simulink model "Multiphase"  (R2018b)
settings: Solver=FixedStepDiscrete  StartTime=0.0  StopTime=10.0  FixedStep=0.05  RelTol=1e-3  EnableMultiTasking=on
undefined symbols (not defined in the file): HRTIM_ADC1R_AD1TAC2, HRTIM_ADC1R_AD1TBC2, HRTIM_ADC1R_AD1TCC2, HRTIM_ADC1R_AD1TDC3, HRTIM_ADC1R_AD1TDC4, HRTIM_TIMERINDEX_TIMER_D, sTimerxRegs
libraries: HRTIMERS_Lib x9, GPIO_Lib x9, REG_Lib x8, STM32_Config_Lib x1
settings Model: Creator=reynaudp  LastModifiedBy=bannou
settings DataIOCC: LimitDataPoints=on  SaveFormat=Array
settings OptimizationCC: DefaultParameterBehavior=Inlined  LifeSpan=1
settings DebuggingCC: SolverPrmCheckMsg=warning  MultiTaskDSMMsg=none  AllowSymbolicDim=off  SFUnexpectedBacktrackingDiag=warning  SFNoUnconditionalDefaultTransitionDiag=warning  SFExecutionAtInitializationDiag=none
settings HardwareCC: ProdBitPerPointer=32  ProdBitPerSizeT=32  ProdBitPerPtrDiffT=32  ProdLargestAtomicInteger=Integer  ProdWordSize=32  ProdHWDeviceType=STMicroelectronics->STM32 32-bit Cortex-M
settings ModelReferenceCC: PropagateSignalLabelsOutOfModel=off
settings SFSimCC: SimUseLocalCustomCode=off  MATLABDynamicMemAlloc=off
settings RTWCC: SystemTargetFile=stm32.tlc  TemplateMakefile=stm32.tmf  Description=stm32 (Embedded Target)  GenerateReport=on  RTWUseLocalCustomCode=off
settings CodeAppCC: IgnoreCustomStorageClasses=off  CustomSymbolStrType=$N$R$M  SimulinkBlockComments=off
settings STFCustomTargetCC: CodeReplacementLibrary=ARM CMSIS SIN COS  ParMdlRefBuildCompliant=on  IncludeMdlTerminateFcn=off  CombineOutputUpdateFcns=on  ERTCustomFileBanners=on  SupportNonFinite=off  SupportComplex=off  SupportContinuousTime=off  SupportNonInlinedSFcns=off  RemoveResetFunc=on  MATLABClassNameForMDSCustomization=Simulink.SoftwareTarget.ERTCustomization  SystemTargetFile=stm32.tlc
settings ERTTargetCC: CodeReplacementLibrary=ARM CMSIS SIN COS  MultiwordLength=2048  CompOptLevelCompliant=off  ConcurrentExecutionCompliant=off  IncludeMdlTerminateFcn=off  SupportNonFinite=off  SupportComplex=off  ModelStepFunctionPrototypeControlCompliant=off  CPPClassGenCompliant=off  UseToolchainInfoCompliant=off  ERTSrcFileBannerTemplate=sourceFileTemplate.cgt  ERTHdrFileBannerTemplate=sourceFileTemplate.cgt  ERTDataSrcFileTemplate=sourceFileTemplate.cgt  ERTDataHdrFileTemplate=sourceFileTemplate.cgt  ERTCustomFileTemplate=customRoutineProcess.tlc  ConvertIfToSwitch=off  SuppressUnreachableDefaultCases=off
settings ConfigComp: CovMetricSettings=dw  CovHtmlReporting=on  CovSaveCumulativeToWorkspaceVar=on  CovSaveSingleToWorkspaceVar=on  CovExternalEMLEnable=off  CovSFcnEnable=off

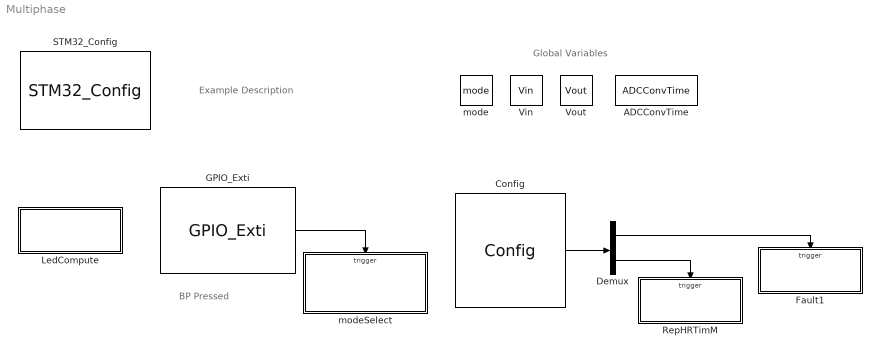
== system Multiphase ==
  note: Example Description
  note: BP Pressed
  note: Global Variables
  ADCConvTime : DataStoreMemory  DataStoreName=ADCConvTime  ReadBeforeWriteMsg=warning  WriteAfterWriteMsg=warning  WriteAfterReadMsg=warning  InitialValue=1152  ShowAdditionalParam=off  OutDataTypeStr=uint32
  Config : HRTIMERS_Lib/Config  currentHRTIM=HRTIM1  NbHRTim=1  HRTIM_Name=HRTIM1  HRTIM_Clock=144000000  TIM_IRQ_F1=on  TIM_IRQ_F2=off  TIM_IRQ_F3=off  TIM_IRQ_F4=off  TIM_IRQ_F5=off  TIM_IRQ_F6=off  TIM_IRQ_SF=off  TIM_IRQ_BMP=off  TIM_IRQ_DLLCALL=off  TIM_IRQ_SYNC=off  TIM_IRQ_BURST_DMA=off  TIM_IRQ_DMA_ERR=off  M_DMA=off  M_IT_global=on  M_Tim_div=MUL32  M_Period=40960  M_PWM_Period=112500  M_Unit1=8192  M_Unit2=16384  M_Unit3=24576  M_Unit4=32768  TIM_IRQ_UPDM=off  TIM_IRQ_REPM=on  TIM_IRQ_COMP1=off  TIM_IRQ_COMP2=off  TIM_IRQ_COMP3=off  TIM_IRQ_COMP4=off  A_Mode=Advanced  A_DMA=off  A_IT_global=off  A_Tim_div=MUL32  A_Period=39807  A_PWM_Period=115759  A_Capture1=off  A_Capture2=off  TA1_Enable=off  TA1_Polarity=HIGH  TA1_Chopper=off  TA2_Enable=on  TA2_Polarity=HIGH  TA2_Chopper=off  A_Unit1=4096  A_Unit2=2048  A_Unit3=37503  A_Unit4=38655  A_Output_Comp1=off  A_Comp_Polarity1=HIGH  A_CompVal1=0  A_Output_Comp2=off  A_Comp_Polarity2=HIGH  A_CompVal2=0  A_Output_PWM1=off  A_Output_Polarity1=HIGH  A_DutyVal1=0  A_DutyIn1=off  A_Output_PWM2=off  A_Output_Polarity2=HIGH  A_DutyVal2=0  A_DutyIn2=off  A_OnePulse1=off  A_OnePulse_Polarity1=HIGH  A_OnePulse_CompVal1=0  A_OnePulse2=off  A_OnePulse_Polarity2=HIGH  A_OnePulse_CompVal2=0  TIM_IRQ_UPDA=off  TIM_IRQ_REPA=off  TIM_IRQ_COMP1A=off  TIM_IRQ_COMP2A=off  TIM_IRQ_COMP3A=off  TIM_IRQ_COMP4A=off  TIM_IRQ_CAPT1A=off  TIM_IRQ_CAPT2A=off  TIM_IRQ_DELA=off  TIM_IRQ_RESET_CPTA=off  TIM_IRQ_OUT1SA=off  TIM_IRQ_OUT1RA=off  TIM_IRQ_OUT2SA=off  TIM_IRQ_OUT2RA=off  B_Mode=Advanced  B_DMA=off  B_IT_global=off  B_Tim_div=MUL32  B_Period=39807  B_PWM_Period=115759  B_Capture1=off  B_Capture2=off  TB1_Enable=on  TB1_Polarity=HIGH  TB1_Chopper=off  TB2_Enable=off  TB2_Polarity=HIGH  TB2_Chopper=off  B_Unit1=4096  B_Unit2=2048  B_Unit3=19327  B_Unit4=18175  B_Output_Comp1=off  B_Comp_Polarity1=HIGH  B_CompVal1=0  B_Output_Comp2=off  B_Comp_Polarity2=HIGH  B_CompVal2=0  B_Output_PWM1=off  B_Output_Polarity1=HIGH  B_DutyVal1=0  B_DutyIn1=off  B_Output_PWM2=off  B_Output_Polarity2=HIGH  B_DutyVal2=0  B_DutyIn2=off  B_OnePulse1=off  B_OnePulse_Polarity1=HIGH  B_OnePulse_CompVal1=0  B_OnePulse2=off  B_OnePulse_Polarity2=HIGH  B_OnePulse_CompVal2=0  TIM_IRQ_UPDB=off  TIM_IRQ_REPB=off  TIM_IRQ_COMP1B=off  TIM_IRQ_COMP2B=off  TIM_IRQ_COMP3B=off  TIM_IRQ_COMP4B=off  TIM_IRQ_CAPT1B=off  TIM_IRQ_CAPT2B=off  TIM_IRQ_DELB=off  TIM_IRQ_RESET_CPTB=off  TIM_IRQ_OUT1SB=off  TIM_IRQ_OUT1RB=off  TIM_IRQ_OUT2SB=off  TIM_IRQ_OUT2RB=off  C_Mode=Advanced  C_DMA=off  C_IT_global=off  C_Tim_div=MUL32  C_Period=39807  C_PWM_Period=115759  C_Capture1=off  C_Capture2=off  TC1_Enable=off  TC1_Polarity=HIGH  TC1_Chopper=off  TC2_Enable=on  TC2_Polarity=HIGH  TC2_Chopper=off  C_Unit1=4096  C_Unit2=2048  C_Unit3=12500  C_Unit4=11348  C_Output_Comp1=off  C_Comp_Polarity1=HIGH  C_CompVal1=0  C_Output_Comp2=off  C_Comp_Polarity2=HIGH  C_CompVal2=0  C_Output_PWM1=off  C_Output_Polarity1=HIGH  C_DutyVal1=0  C_DutyIn1=off  C_Output_PWM2=off  C_Output_Polarity2=HIGH  C_DutyVal2=0  C_DutyIn2=off  C_OnePulse1=off  C_OnePulse_Polarity1=HIGH  C_OnePulse_CompVal1=0  C_OnePulse2=off  C_OnePulse_Polarity2=HIGH  C_OnePulse_CompVal2=0  TIM_IRQ_UPDC=off  TIM_IRQ_REPC=off  TIM_IRQ_COMP1C=off  TIM_IRQ_COMP2C=off  TIM_IRQ_COMP3C=off  TIM_IRQ_COMP4C=off  TIM_IRQ_CAPT1C=off  TIM_IRQ_CAPT2C=off  TIM_IRQ_DELC=off  TIM_IRQ_RESET_CPTC=off  TIM_IRQ_OUT1SC=off  TIM_IRQ_OUT1RC=off  TIM_IRQ_OUT2SC=off  TIM_IRQ_OUT2RC=off  D_Mode=Advanced  D_DMA=off  D_IT_global=off  D_Tim_div=MUL32  D_Period=39807  D_PWM_Period=115759  D_Capture1=off  D_Capture2=off  TD1_Enable=on  TD1_Polarity=HIGH  TD1_Chopper=off  TD2_Enable=on  TD2_Polarity=HIGH  TD2_Chopper=off  D_Unit1=4096  D_Unit2=12288  D_Unit3=2048  D_Unit4=10240  D_Output_Comp1=off  D_Comp_Polarity1=HIGH  D_CompVal1=0  D_Output_Comp2=off  D_Comp_Polarity2=HIGH  D_CompVal2=0  D_Output_PWM1=off  D_Output_Polarity1=HIGH  D_DutyVal1=0  D_DutyIn1=off  D_Output_PWM2=off  D_Output_Polarity2=HIGH  D_DutyVal2=0  D_DutyIn2=off  D_OnePulse1=off  D_OnePulse_Polarity1=HIGH  D_OnePulse_CompVal1=0  D_OnePulse2=off  D_OnePulse_Polarity2=HIGH  D_OnePulse_CompVal2=0  TIM_IRQ_UPDD=off  TIM_IRQ_REPD=off  TIM_IRQ_COMP1D=off  TIM_IRQ_COMP2D=off  TIM_IRQ_COMP3D=off  TIM_IRQ_COMP4D=off  TIM_IRQ_CAPT1D=off  TIM_IRQ_CAPT2D=off  TIM_IRQ_DELD=off  TIM_IRQ_RESET_CPTD=off  TIM_IRQ_OUT1SD=off  TIM_IRQ_OUT1RD=off  TIM_IRQ_OUT2SD=off  TIM_IRQ_OUT2RD=off  E_Mode=Advanced  E_DMA=off  E_IT_global=off  E_Tim_div=MUL32  E_Period=0  E_PWM_Period=Inf  E_Capture1=off  E_Capture2=off  TE1_Enable=off  TE1_Polarity=HIGH  TE1_Chopper=off  TE2_Enable=off  TE2_Polarity=HIGH  TE2_Chopper=off  E_Unit1=0  E_Unit2=0  E_Unit3=0  E_Unit4=0  E_Output_Comp1=off  E_Comp_Polarity1=HIGH  E_CompVal1=0  E_Output_Comp2=off  E_Comp_Polarity2=HIGH  E_CompVal2=0  E_Output_PWM1=off  E_Output_Polarity1=HIGH  E_DutyVal1=0  E_DutyIn1=off  E_Output_PWM2=off  E_Output_Polarity2=HIGH  E_DutyVal2=0  E_DutyIn2=off  E_OnePulse1=off  E_OnePulse_Polarity1=HIGH  E_OnePulse_CompVal1=0  E_OnePulse2=off  E_OnePulse_Polarity2=HIGH  E_OnePulse_CompVal2=0  TIM_IRQ_UPDE=off  TIM_IRQ_REPE=off  TIM_IRQ_COMP1E=off  TIM_IRQ_COMP2E=off  TIM_IRQ_COMP3E=off  TIM_IRQ_COMP4E=off  TIM_IRQ_CAPT1E=off  TIM_IRQ_CAPT2E=off  TIM_IRQ_DELE=off  TIM_IRQ_RESET_CPTE=off  TIM_IRQ_OUT1SE=off  TIM_IRQ_OUT1RE=off  TIM_IRQ_OUT2SE=off  TIM_IRQ_OUT2RE=off  F_Mode=Advanced  F_DMA=off  F_IT_global=off  F_Tim_div=MUL32  F_Period=0  F_PWM_Period=Inf  F_Capture1=off  F_Capture2=off  TF1_Enable=off  TF1_Polarity=HIGH  TF1_Chopper=off  TF2_Enable=off  TF2_Polarity=HIGH  TF2_Chopper=off  F_Unit1=0  F_Unit2=0  F_Unit3=0  F_Unit4=0  F_Output_Comp1=off  F_Comp_Polarity1=HIGH  F_CompVal1=0  F_Output_Comp2=off  F_Comp_Polarity2=HIGH  F_CompVal2=0  F_Output_PWM1=off  F_Output_Polarity1=HIGH  F_DutyVal1=0  F_DutyIn1=off  F_Output_PWM2=off  F_Output_Polarity2=HIGH  F_DutyVal2=0  F_DutyIn2=off  F_OnePulse1=off  F_OnePulse_Polarity1=HIGH  F_OnePulse_CompVal1=0  F_OnePulse2=off  F_OnePulse_Polarity2=HIGH  F_OnePulse_CompVal2=0  TIM_IRQ_UPDF=off  TIM_IRQ_REPF=off  TIM_IRQ_COMP1F=off  TIM_IRQ_COMP2F=off  TIM_IRQ_COMP3F=off  TIM_IRQ_COMP4F=off  TIM_IRQ_CAPT1F=off  TIM_IRQ_CAPT2F=off  TIM_IRQ_DELF=off  TIM_IRQ_RESET_CPTF=off  TIM_IRQ_OUT1SF=off  TIM_IRQ_OUT1RF=off  TIM_IRQ_OUT2SF=off  TIM_IRQ_OUT2RF=off  M_Used=on  A_Used=on  B_Used=on  C_Used=on  D_Used=on  E_Used=off  F_Used=off
      settings: SourceProductName=Target Support Package - STM32 Adapter
  Demux : Demux  Outputs=2
  Fault1 : Subsystem  TreatAsAtomicUnit=on
  GPIO_Exti : GPIO_Lib/GPIO_Exti  Priority=0  Port_name=GPIOA  Pin_0=on  Pin_1=off  Pin_2=off  Pin_3=off  Pin_4=off  Pin_5=off  Pin_6=off  Pin_7=off  Pin_8=off  Pin_9=off  Pin_10=off  Pin_11=off  Pin_12=off  Pin_13=off  Pin_14=off  Pin_15=off  PinList=GPIOA0
      settings: SourceProductName=Target Support Package - STM32 Adapter
  LedCompute : Subsystem
  RepHRTimM : Subsystem  TreatAsAtomicUnit=on
  STM32_Config : STM32_Config_Lib/STM32_Config  Priority=0  Project_Path=.\  Config_File=Multiphase.ioc  MCU_Name=STM32F334C8Tx
      settings: SourceProductName=Target Support Package - STM32 Adapter
  Vin : DataStoreMemory  DataStoreName=Vin  ReadBeforeWriteMsg=warning  WriteAfterWriteMsg=warning  WriteAfterReadMsg=warning  ShowAdditionalParam=off  OutMin=0  OutMax=5000  OutDataTypeStr=uint32
  Vout : DataStoreMemory  DataStoreName=Vout  ReadBeforeWriteMsg=warning  WriteAfterWriteMsg=warning  WriteAfterReadMsg=warning  ShowAdditionalParam=off  OutMin=0  OutDataTypeStr=uint32
  mode : DataStoreMemory  DataStoreName=mode  ReadBeforeWriteMsg=warning  WriteAfterWriteMsg=warning  WriteAfterReadMsg=warning  InitialValue=6  ShowAdditionalParam=off  OutMin=0  OutMax=12  OutDataTypeStr=uint8
  modeSelect : Subsystem  TreatAsAtomicUnit=on
  wires:
  GPIO_Exti/1 -> modeSelect/Trigger
  Config/1 -> Demux/1
  Demux/1 -> Fault1/Trigger
  Demux/2 -> RepHRTimM/Trigger

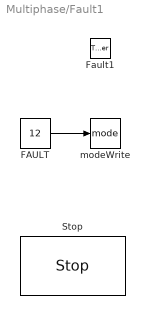
== system Multiphase/Fault1 ==
  Fault1 : TriggerPort  TriggerType=function-call  VariantControl=Variant
  FAULT : Constant  Value=12  OutDataTypeStr=uint8
  Stop : HRTIMERS_Lib/Stop  currentHRTIM=HRTIM1  NbHRTim=1  HRTIM_Name=HRTIM1  TA1_Stop=off  TA2_Stop=on  TB1_Stop=on  TB2_Stop=off  TC1_Stop=off  TC2_Stop=on  TD1_Stop=on  TD2_Stop=on  TE1_Stop=off  TE2_Stop=off  TF1_Stop=off  TF2_Stop=off
      settings: SourceProductName=Target Support Package - STM32 Adapter
  modeWrite : DataStoreWrite  DataStoreName=mode
  wires:
  FAULT/1 -> modeWrite/1

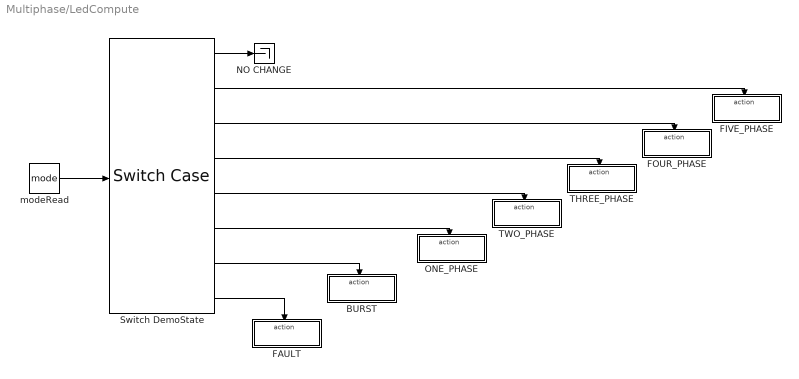
== system Multiphase/LedCompute ==
  BURST : Subsystem  TreatAsAtomicUnit=on
  FAULT : Subsystem  TreatAsAtomicUnit=on
  FIVE_PHASE : Subsystem  TreatAsAtomicUnit=on
  FOUR_PHASE : Subsystem  TreatAsAtomicUnit=on
  NO CHANGE : Terminator
  ONE_PHASE : Subsystem  TreatAsAtomicUnit=on
  Switch DemoState : SwitchCase  CaseConditions={[0,5],6,7,8,9,10,11,12}  ShowDefaultCase=off
  THREE_PHASE : Subsystem  TreatAsAtomicUnit=on
  TWO_PHASE : Subsystem  TreatAsAtomicUnit=on
  modeRead : DataStoreRead  DialogController=Simulink.DDGSource  DataStoreName=mode
  wires:
  modeRead/1 -> Switch DemoState/1
  Switch DemoState/2 -> FIVE_PHASE/Action
  Switch DemoState/3 -> FOUR_PHASE/Action
  Switch DemoState/4 -> THREE_PHASE/Action
  Switch DemoState/5 -> TWO_PHASE/Action
  Switch DemoState/6 -> ONE_PHASE/Action
  Switch DemoState/7 -> BURST/Action
  Switch DemoState/8 -> FAULT/Action
  Switch DemoState/1 -> NO CHANGE/1

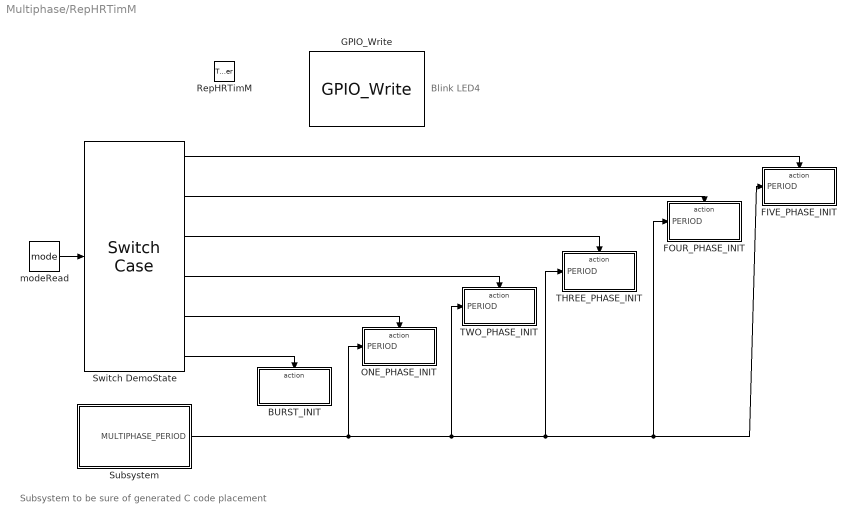
== system Multiphase/RepHRTimM ==
  note: Blink LED4
  note: Subsystem to be sure of generated C code placement
  RepHRTimM : TriggerPort  TriggerType=function-call  VariantControl=Variant
  BURST_INIT : Subsystem  TreatAsAtomicUnit=on
  FIVE_PHASE_INIT : Subsystem  TreatAsAtomicUnit=on
  FOUR_PHASE_INIT : Subsystem  TreatAsAtomicUnit=on
  GPIO_Write : GPIO_Lib/GPIO_Write  Port_name=GPIOB  Pin0=off  Toggle_Pin0=off  Pin1=off  Toggle_Pin1=off  Pin2=off  Toggle_Pin2=off  Pin3=off  Toggle_Pin3=off  Pin4=off  Toggle_Pin4=off  Pin5=off  Toggle_Pin5=off  Pin6=off  Toggle_Pin6=off  Pin7=off  Toggle_Pin7=off  Pin8=on  Toggle_Pin8=on  Pin9=off  Toggle_Pin9=off  Pin10=off  Toggle_Pin10=off  Pin11=off  Toggle_Pin11=off  Pin12=off  Toggle_Pin12=off  Pin13=off  Toggle_Pin13=off  Pin14=off  Toggle_Pin14=off  Pin15=off  Toggle_Pin15=off  PinList="GPIOB6  7  8  9"
      settings: SourceProductName=Target Support Package - STM32 Adapter
  ONE_PHASE_INIT : Subsystem  TreatAsAtomicUnit=on
  Subsystem : Subsystem  TreatAsAtomicUnit=on
      settings: RTWSystemCode=Inline
  Switch DemoState : SwitchCase  Priority=0  CaseConditions={0,1,2,3,4,5}  ShowDefaultCase=off
  THREE_PHASE_INIT : Subsystem  TreatAsAtomicUnit=on
  TWO_PHASE_INIT : Subsystem  TreatAsAtomicUnit=on
  modeRead : DataStoreRead  DataStoreName=mode
  wires:
  modeRead/1 -> Switch DemoState/1
  Switch DemoState/1 -> FIVE_PHASE_INIT/Action
  Switch DemoState/2 -> FOUR_PHASE_INIT/Action
  Switch DemoState/3 -> THREE_PHASE_INIT/Action
  Switch DemoState/4 -> TWO_PHASE_INIT/Action
  Switch DemoState/5 -> ONE_PHASE_INIT/Action
  Switch DemoState/6 -> BURST_INIT/Action
  Subsystem/1(MULTIPHASE_PERIOD) -> ONE_PHASE_INIT/1(PERIOD), TWO_PHASE_INIT/1(PERIOD), THREE_PHASE_INIT/1(PERIOD), FOUR_PHASE_INIT/1(PERIOD), FIVE_PHASE_INIT/1(PERIOD)

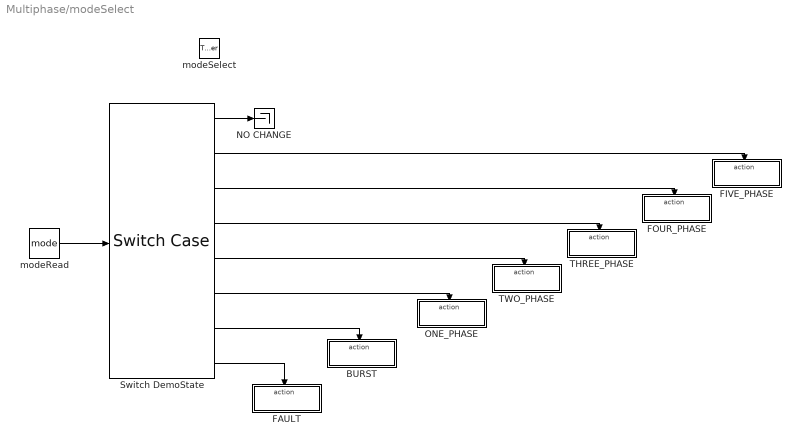
== system Multiphase/modeSelect ==
  modeSelect : TriggerPort  TriggerType=function-call  VariantControl=Variant
  BURST : Subsystem  TreatAsAtomicUnit=on
  FAULT : Subsystem  TreatAsAtomicUnit=on
  FIVE_PHASE : Subsystem  TreatAsAtomicUnit=on
  FOUR_PHASE : Subsystem  TreatAsAtomicUnit=on
  NO CHANGE : Terminator
  ONE_PHASE : Subsystem  TreatAsAtomicUnit=on
  Switch DemoState : SwitchCase  CaseConditions={[0,5],6,7,8,9,10,11,12}  ShowDefaultCase=off
  THREE_PHASE : Subsystem  TreatAsAtomicUnit=on
  TWO_PHASE : Subsystem  TreatAsAtomicUnit=on
  modeRead : DataStoreRead  DialogController=Simulink.DDGSource  DataStoreName=mode
  wires:
  modeRead/1 -> Switch DemoState/1
  Switch DemoState/2 -> FIVE_PHASE/Action
  Switch DemoState/3 -> FOUR_PHASE/Action
  Switch DemoState/4 -> THREE_PHASE/Action
  Switch DemoState/5 -> TWO_PHASE/Action
  Switch DemoState/6 -> ONE_PHASE/Action
  Switch DemoState/7 -> BURST/Action
  Switch DemoState/8 -> FAULT/Action
  Switch DemoState/1 -> NO CHANGE/1

== system Multiphase/LedCompute/BURST ==
  BURST : ActionPort  ActionType=case
  GPIO_Write : GPIO_Lib/GPIO_Write  Port_name=GPIOB  Pin0=off  Toggle_Pin0=off  Pin1=off  Toggle_Pin1=off  Pin2=off  Toggle_Pin2=off  Pin3=off  Toggle_Pin3=off  Pin4=off  Toggle_Pin4=off  Pin5=off  Toggle_Pin5=off  Pin6=off  Toggle_Pin6=off  Pin7=on  Toggle_Pin7=on  Pin8=off  Toggle_Pin8=off  Pin9=on  Toggle_Pin9=on  Pin10=off  Toggle_Pin10=off  Pin11=off  Toggle_Pin11=off  Pin12=off  Toggle_Pin12=off  Pin13=off  Toggle_Pin13=off  Pin14=off  Toggle_Pin14=off  Pin15=off  Toggle_Pin15=off  PinList="GPIOB6  7  8  9"
      settings: SourceProductName=Target Support Package - STM32 Adapter

== system Multiphase/LedCompute/FAULT ==
  FAULT : ActionPort  ActionType=case
  GPIO_Write : GPIO_Lib/GPIO_Write  Port_name=GPIOB  Pin0=off  Toggle_Pin0=off  Pin1=off  Toggle_Pin1=off  Pin2=off  Toggle_Pin2=off  Pin3=off  Toggle_Pin3=off  Pin4=off  Toggle_Pin4=off  Pin5=off  Toggle_Pin5=off  Pin6=on  Toggle_Pin6=on  Pin7=on  Toggle_Pin7=off  Pin8=off  Toggle_Pin8=off  Pin9=on  Toggle_Pin9=off  Pin10=off  Toggle_Pin10=off  Pin11=off  Toggle_Pin11=off  Pin12=off  Toggle_Pin12=off  Pin13=off  Toggle_Pin13=off  Pin14=off  Toggle_Pin14=off  Pin15=off  Toggle_Pin15=off  PinList="GPIOB6  7  8  9"
      settings: SourceProductName=Target Support Package - STM32 Adapter
  LED_OFF : Constant  Value=0
  wires:
  LED_OFF/1 -> GPIO_Write/2, GPIO_Write/1

== system Multiphase/LedCompute/FIVE_PHASE ==
  FIVE_PHASE : ActionPort  ActionType=case
  GPIO_Write : GPIO_Lib/GPIO_Write  Port_name=GPIOB  Pin0=off  Toggle_Pin0=off  Pin1=off  Toggle_Pin1=off  Pin2=off  Toggle_Pin2=off  Pin3=off  Toggle_Pin3=off  Pin4=off  Toggle_Pin4=off  Pin5=off  Toggle_Pin5=off  Pin6=on  Toggle_Pin6=off  Pin7=on  Toggle_Pin7=off  Pin8=off  Toggle_Pin8=off  Pin9=on  Toggle_Pin9=on  Pin10=off  Toggle_Pin10=off  Pin11=off  Toggle_Pin11=off  Pin12=off  Toggle_Pin12=off  Pin13=off  Toggle_Pin13=off  Pin14=off  Toggle_Pin14=off  Pin15=off  Toggle_Pin15=off  PinList="GPIOB6  7  8  9"
      settings: SourceProductName=Target Support Package - STM32 Adapter
  LED_OFF : Constant  Value=0
  wires:
  LED_OFF/1 -> GPIO_Write/2, GPIO_Write/1

== system Multiphase/LedCompute/FOUR_PHASE ==
  FOUR_PHASE : ActionPort  ActionType=case
  GPIO_Write : GPIO_Lib/GPIO_Write  Port_name=GPIOB  Pin0=off  Toggle_Pin0=off  Pin1=off  Toggle_Pin1=off  Pin2=off  Toggle_Pin2=off  Pin3=off  Toggle_Pin3=off  Pin4=off  Toggle_Pin4=off  Pin5=off  Toggle_Pin5=off  Pin6=off  Toggle_Pin6=off  Pin7=on  Toggle_Pin7=on  Pin8=off  Toggle_Pin8=off  Pin9=on  Toggle_Pin9=off  Pin10=off  Toggle_Pin10=off  Pin11=off  Toggle_Pin11=off  Pin12=off  Toggle_Pin12=off  Pin13=off  Toggle_Pin13=off  Pin14=off  Toggle_Pin14=off  Pin15=off  Toggle_Pin15=off  PinList="GPIOB6  7  8  9"
      settings: SourceProductName=Target Support Package - STM32 Adapter
  LED_OFF : Constant  Value=0
  wires:
  LED_OFF/1 -> GPIO_Write/1

== system Multiphase/LedCompute/ONE_PHASE ==
  ONE_PHASE : ActionPort  ActionType=case
  GPIO_Write : GPIO_Lib/GPIO_Write  Port_name=GPIOB  Pin0=off  Toggle_Pin0=off  Pin1=off  Toggle_Pin1=off  Pin2=off  Toggle_Pin2=off  Pin3=off  Toggle_Pin3=off  Pin4=off  Toggle_Pin4=off  Pin5=off  Toggle_Pin5=off  Pin6=off  Toggle_Pin6=off  Pin7=on  Toggle_Pin7=off  Pin8=off  Toggle_Pin8=off  Pin9=on  Toggle_Pin9=off  Pin10=off  Toggle_Pin10=off  Pin11=off  Toggle_Pin11=off  Pin12=off  Toggle_Pin12=off  Pin13=off  Toggle_Pin13=off  Pin14=off  Toggle_Pin14=off  Pin15=off  Toggle_Pin15=off  PinList="GPIOB6  7  8  9"
      settings: SourceProductName=Target Support Package - STM32 Adapter
  LED_ON : Constant
  wires:
  LED_ON/1 -> GPIO_Write/1, GPIO_Write/2

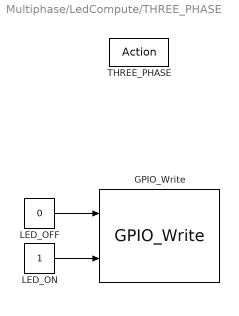
== system Multiphase/LedCompute/THREE_PHASE ==
  THREE_PHASE : ActionPort  ActionType=case
  GPIO_Write : GPIO_Lib/GPIO_Write  Port_name=GPIOB  Pin0=off  Toggle_Pin0=off  Pin1=off  Toggle_Pin1=off  Pin2=off  Toggle_Pin2=off  Pin3=off  Toggle_Pin3=off  Pin4=off  Toggle_Pin4=off  Pin5=off  Toggle_Pin5=off  Pin6=off  Toggle_Pin6=off  Pin7=on  Toggle_Pin7=off  Pin8=off  Toggle_Pin8=off  Pin9=on  Toggle_Pin9=off  Pin10=off  Toggle_Pin10=off  Pin11=off  Toggle_Pin11=off  Pin12=off  Toggle_Pin12=off  Pin13=off  Toggle_Pin13=off  Pin14=off  Toggle_Pin14=off  Pin15=off  Toggle_Pin15=off  PinList="GPIOB6  7  8  9"
      settings: SourceProductName=Target Support Package - STM32 Adapter
  LED_OFF : Constant  Value=0
  LED_ON : Constant
  wires:
  LED_OFF/1 -> GPIO_Write/1
  LED_ON/1 -> GPIO_Write/2

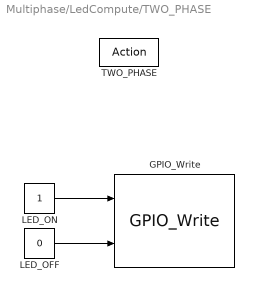
== system Multiphase/LedCompute/TWO_PHASE ==
  TWO_PHASE : ActionPort  ActionType=case
  GPIO_Write : GPIO_Lib/GPIO_Write  Port_name=GPIOB  Pin0=off  Toggle_Pin0=off  Pin1=off  Toggle_Pin1=off  Pin2=off  Toggle_Pin2=off  Pin3=off  Toggle_Pin3=off  Pin4=off  Toggle_Pin4=off  Pin5=off  Toggle_Pin5=off  Pin6=off  Toggle_Pin6=off  Pin7=on  Toggle_Pin7=off  Pin8=off  Toggle_Pin8=off  Pin9=on  Toggle_Pin9=off  Pin10=off  Toggle_Pin10=off  Pin11=off  Toggle_Pin11=off  Pin12=off  Toggle_Pin12=off  Pin13=off  Toggle_Pin13=off  Pin14=off  Toggle_Pin14=off  Pin15=off  Toggle_Pin15=off  PinList="GPIOB6  7  8  9"
      settings: SourceProductName=Target Support Package - STM32 Adapter
  LED_OFF : Constant  Value=0
  LED_ON : Constant
  wires:
  LED_OFF/1 -> GPIO_Write/2
  LED_ON/1 -> GPIO_Write/1

== system Multiphase/RepHRTimM/BURST_INIT ==
  Action Port : ActionPort  ActionType=case
  BURST : Constant  Value=11  OutDataTypeStr=uint8
  REG_Access1 : REG_Lib/REG_Access  Peripheral=HRTIM1  RegName=sCommonRegs.BMCR  RegRead=off  RegWrite=on  RegValueIn=off  RegValue=HRTIM_BMCR_BME  RegEqual=off  RegAnd=off  RegOr=on  RegComplement=off  RegComments=Enable Burst mode (will start on next Master timer period)  currentPeriph=HRTIM1
      settings: SourceProductName=Target Support Package - STM32 Adapter
  modeWrite : DataStoreWrite  DataStoreName=mode
  wires:
  BURST/1 -> modeWrite/1

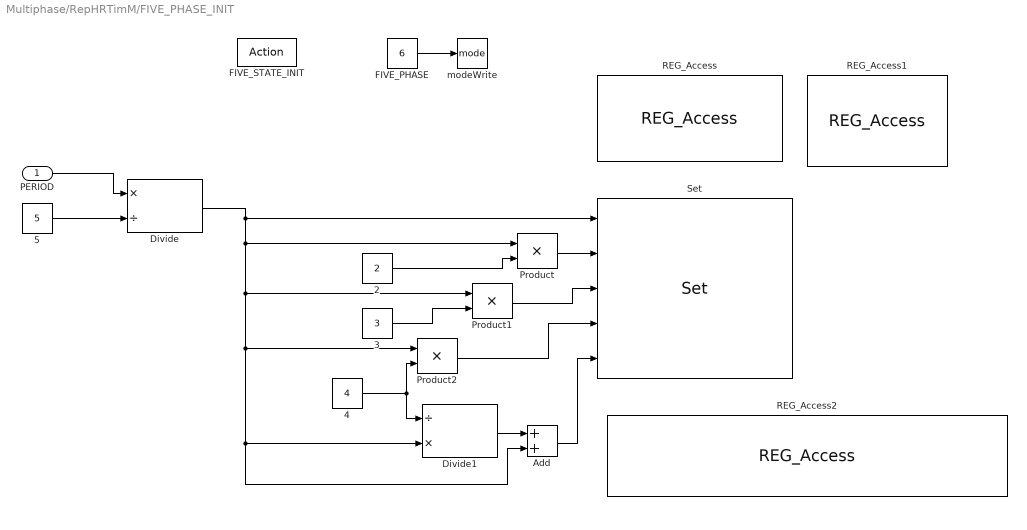
== system Multiphase/RepHRTimM/FIVE_PHASE_INIT ==
  PERIOD : Inport
  FIVE_STATE_INIT : ActionPort  ActionType=case
  2 : Constant  Value=2  OutDataTypeStr=uint32
  3 : Constant  Value=3  OutDataTypeStr=uint32
  4 : Constant  Value=4  OutDataTypeStr=uint32
  5 : Constant  Value=5  OutDataTypeStr=uint32
  Add : Sum  OutDataTypeStr=uint32  InputSameDT=on
  Divide : Product  Inputs=*/  OutDataTypeStr=uint32  InputSameDT=on
  Divide1 : Product  Inputs=/*  OutDataTypeStr=uint32  InputSameDT=on
  FIVE_PHASE : Constant  Value=6  OutDataTypeStr=uint8
  Product : Product  OutDataTypeStr=uint32  InputSameDT=on
  Product1 : Product  OutDataTypeStr=uint32  InputSameDT=on
  Product2 : Product  OutDataTypeStr=uint32  InputSameDT=on
  REG_Access : REG_Lib/REG_Access  Peripheral=HRTIM1  RegName=sCommonRegs.ADC1R  RegRead=off  RegWrite=on  RegValueIn=off  RegValue=HRTIM_ADC1R_AD1TAC2+HRTIM_ADC1R_AD1TBC2+HRTIM_ADC1R_AD1TCC2+HRTIM_ADC1R_AD1TDC3+HRTIM_ADC1R_AD1TDC4  RegEqual=on  RegAnd=off  RegOr=off  RegComplement=off  RegComments=Reconfigure triggers for 5 conversions  currentPeriph=HRTIM1
      settings: SourceProductName=Target Support Package - STM32 Adapter
  REG_Access1 : REG_Lib/REG_Access  Peripheral=HRTIM1  RegName=sCommonRegs.BMCR  RegRead=off  RegWrite=on  RegValueIn=off  RegValue=HRTIM_BMCR_BME  RegEqual=off  RegAnd=on  RegOr=off  RegComplement=on  RegComments=Disable burst mode  currentPeriph=HRTIM1
      settings: SourceProductName=Target Support Package - STM32 Adapter
  REG_Access2 : REG_Lib/REG_Access  Peripheral=HRTIM1  RegName=sTimerxRegs[HRTIM_TIMERINDEX_TIMER_D].SETx2R  RegRead=off  RegWrite=on  RegValueIn=off  RegValue=HRTIM_OUTPUTSET_MASTERCMP4  RegEqual=on  RegAnd=off  RegOr=off  RegComplement=off  RegComments=Restore waveform generation for TD2 (CMP4 is used as ADC trigger in case of single-phase)  currentPeriph=HRTIM1
      settings: SourceProductName=Target Support Package - STM32 Adapter
  Set : HRTIMERS_Lib/Set  currentHRTIM=HRTIM1  NbHRTim=1  HRTIM_Name=HRTIM1  M_Used=on  M_Comp1_In=on  M_Comp1=0  M_Comp2_In=on  M_Comp2=0  M_Comp3_In=on  M_Comp3=0  M_Comp4_In=on  M_Comp4=0  A_Used=on  A_Comp1_In=off  A_Comp1=0  A_Comp2_In=off  A_Comp2=0  A_Comp3_In=off  A_Comp3=0  A_Comp4_In=off  A_Comp4=0  B_Used=on  B_Comp1_In=off  B_Comp1=0  B_Comp2_In=off  B_Comp2=0  B_Comp3_In=off  B_Comp3=0  B_Comp4_In=off  B_Comp4=0  C_Used=on  C_Comp1_In=off  C_Comp1=0  C_Comp2_In=off  C_Comp2=0  C_Comp3_In=off  C_Comp3=0  C_Comp4_In=off  C_Comp4=0  D_Used=on  D_Comp1_In=off  D_Comp1=0  D_Comp2_In=off  D_Comp2=0  D_Comp3_In=off  D_Comp3=0  D_Comp4_In=on  D_Comp4=0  E_Used=off  E_Comp1_In=off  E_Comp1=0  E_Comp2_In=off  E_Comp2=0  E_Comp3_In=off  E_Comp3=0  E_Comp4_In=off  E_Comp4=0  F_Used=off  F_Comp1_In=off  F_Comp1=0  F_Comp2_In=off  F_Comp2=0  F_Comp3_In=off  F_Comp3=0  F_Comp4_In=off  F_Comp4=0
      settings: SourceProductName=Target Support Package - STM32 Adapter
  modeWrite : DataStoreWrite  DataStoreName=mode
  wires:
  FIVE_PHASE/1 -> modeWrite/1
  PERIOD/1 -> Divide/1
  5/1 -> Divide/2
  Divide/1 -> Product/1, Product1/1, Product2/1, Divide1/2, Add/2, Set/1
  Product/1 -> Set/2
  Product1/1 -> Set/3
  Product2/1 -> Set/4
  2/1 -> Product/2
  3/1 -> Product1/2
  4/1 -> Product2/2, Divide1/1
  Divide1/1 -> Add/1
  Add/1 -> Set/5

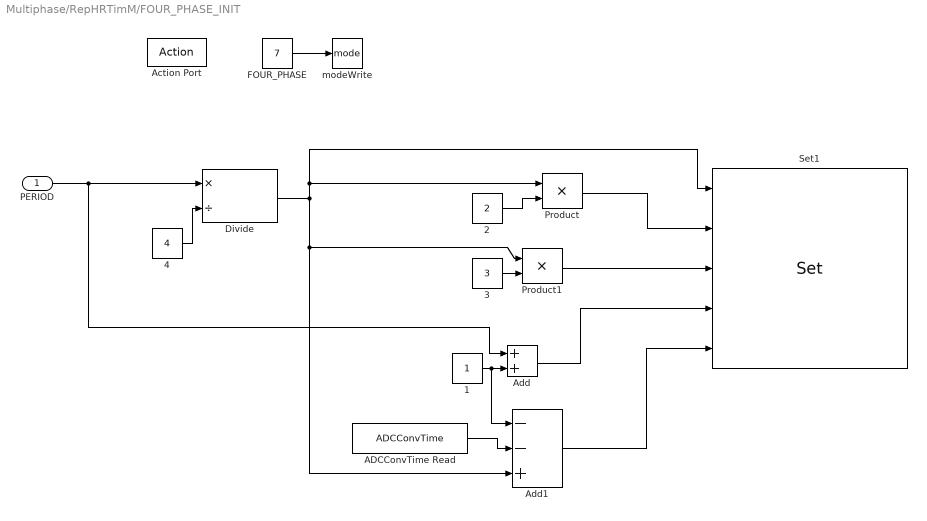
== system Multiphase/RepHRTimM/FOUR_PHASE_INIT ==
  PERIOD : Inport
  Action Port : ActionPort  ActionType=case
  1 : Constant  OutDataTypeStr=uint32
  2 : Constant  Value=2  OutDataTypeStr=uint32
  3 : Constant  Value=3  OutDataTypeStr=uint32
  4 : Constant  Value=4  OutDataTypeStr=uint32
  ADCConvTime Read : DataStoreRead  DataStoreName=ADCConvTime
  Add : Sum  AccumDataTypeStr=uint32  InputSameDT=on
  Add1 : Sum  Inputs=--+  AccumDataTypeStr=uint32  InputSameDT=on
  Divide : Product  Inputs=*/  OutDataTypeStr=uint32  InputSameDT=on
  FOUR_PHASE : Constant  Value=7  OutDataTypeStr=uint8
  Product : Product  OutDataTypeStr=uint32  InputSameDT=on
  Product1 : Product  OutDataTypeStr=uint32  InputSameDT=on
  Set1 : HRTIMERS_Lib/Set  currentHRTIM=HRTIM1  NbHRTim=1  HRTIM_Name=HRTIM1  M_Used=on  M_Comp1_In=on  M_Comp1=0  M_Comp2_In=on  M_Comp2=0  M_Comp3_In=on  M_Comp3=0  M_Comp4_In=on  M_Comp4=0  A_Used=on  A_Comp1_In=off  A_Comp1=0  A_Comp2_In=off  A_Comp2=0  A_Comp3_In=off  A_Comp3=0  A_Comp4_In=off  A_Comp4=0  B_Used=on  B_Comp1_In=off  B_Comp1=0  B_Comp2_In=off  B_Comp2=0  B_Comp3_In=off  B_Comp3=0  B_Comp4_In=off  B_Comp4=0  C_Used=on  C_Comp1_In=off  C_Comp1=0  C_Comp2_In=off  C_Comp2=0  C_Comp3_In=off  C_Comp3=0  C_Comp4_In=off  C_Comp4=0  D_Used=on  D_Comp1_In=off  D_Comp1=0  D_Comp2_In=off  D_Comp2=0  D_Comp3_In=off  D_Comp3=0  D_Comp4_In=on  D_Comp4=0  E_Used=off  E_Comp1_In=off  E_Comp1=0  E_Comp2_In=off  E_Comp2=0  E_Comp3_In=off  E_Comp3=0  E_Comp4_In=off  E_Comp4=0  F_Used=off  F_Comp1_In=off  F_Comp1=0  F_Comp2_In=off  F_Comp2=0  F_Comp3_In=off  F_Comp3=0  F_Comp4_In=off  F_Comp4=0
      settings: SourceProductName=Target Support Package - STM32 Adapter
  modeWrite : DataStoreWrite  DataStoreName=mode
  wires:
  FOUR_PHASE/1 -> modeWrite/1
  PERIOD/1 -> Add/1, Divide/1
  4/1 -> Divide/2
  Divide/1 -> Product/1, Set1/1, Add1/3, Product1/1
  Product/1 -> Set1/2
  2/1 -> Product/2
  3/1 -> Product1/2
  Product1/1 -> Set1/3
  1/1 -> Add1/1, Add/2
  Add/1 -> Set1/4
  ADCConvTime Read/1 -> Add1/2
  Add1/1 -> Set1/5

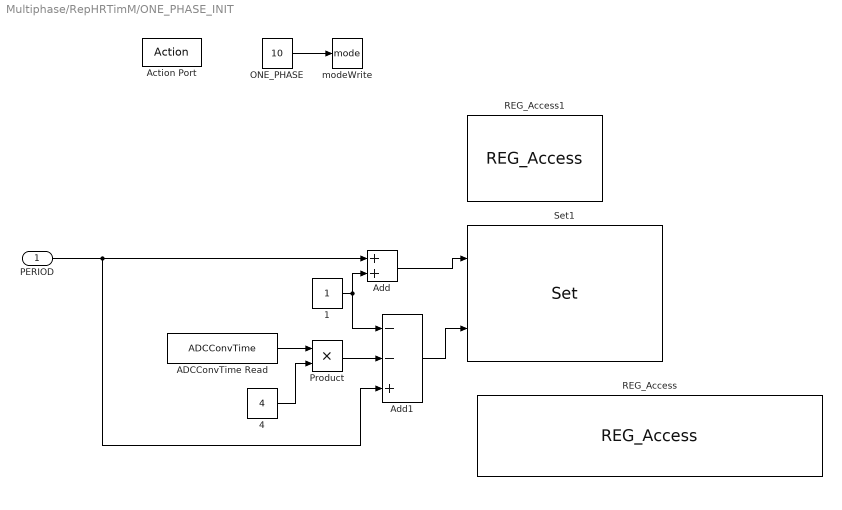
== system Multiphase/RepHRTimM/ONE_PHASE_INIT ==
  PERIOD : Inport
  Action Port : ActionPort  ActionType=case
  1 : Constant  OutDataTypeStr=uint32
  4 : Constant  Value=4  OutDataTypeStr=uint32
  ADCConvTime Read : DataStoreRead  DataStoreName=ADCConvTime
  Add : Sum  OutDataTypeStr=uint32  InputSameDT=on
  Add1 : Sum  Inputs=--+  OutDataTypeStr=uint32  InputSameDT=on
  ONE_PHASE : Constant  Value=10  OutDataTypeStr=uint8
  Product : Product  OutDataTypeStr=uint32
  REG_Access : REG_Lib/REG_Access  Peripheral=HRTIM1  RegName=sCommonRegs.ADC1R  RegRead=off  RegWrite=on  RegValueIn=off  RegValue=<binary blob, 181 chars, not shown>  RegEqual=on  RegAnd=off  RegOr=off  RegComplement=off  RegComments=Reconfigure ADC triggers for a dummy 2nd, 3rd, 4th and 5th conversion  currentPeriph=HRTIM1
      settings: SourceProductName=Target Support Package - STM32 Adapter
  REG_Access1 : REG_Lib/REG_Access  Peripheral=HRTIM1  RegName=sTimerxRegs[HRTIM_TIMERINDEX_TIMER_D].SETx2R  RegRead=off  RegWrite=on  RegValueIn=off  RegValue=0  RegEqual=on  RegAnd=off  RegOr=off  RegComplement=off  currentPeriph=HRTIM1
      settings: SourceProductName=Target Support Package - STM32 Adapter
  Set1 : HRTIMERS_Lib/Set  currentHRTIM=HRTIM1  NbHRTim=1  HRTIM_Name=HRTIM1  M_Used=on  M_Comp1_In=on  M_Comp1=0  M_Comp2_In=off  M_Comp2=0  M_Comp3_In=off  M_Comp3=0  M_Comp4_In=on  M_Comp4=0  A_Used=on  A_Comp1_In=off  A_Comp1=0  A_Comp2_In=off  A_Comp2=0  A_Comp3_In=off  A_Comp3=0  A_Comp4_In=off  A_Comp4=0  B_Used=on  B_Comp1_In=off  B_Comp1=0  B_Comp2_In=off  B_Comp2=0  B_Comp3_In=off  B_Comp3=0  B_Comp4_In=off  B_Comp4=0  C_Used=on  C_Comp1_In=off  C_Comp1=0  C_Comp2_In=off  C_Comp2=0  C_Comp3_In=off  C_Comp3=0  C_Comp4_In=off  C_Comp4=0  D_Used=on  D_Comp1_In=off  D_Comp1=0  D_Comp2_In=off  D_Comp2=0  D_Comp3_In=off  D_Comp3=0  D_Comp4_In=off  D_Comp4=0  E_Used=off  E_Comp1_In=off  E_Comp1=0  E_Comp2_In=off  E_Comp2=0  E_Comp3_In=off  E_Comp3=0  E_Comp4_In=off  E_Comp4=0  F_Used=off  F_Comp1_In=off  F_Comp1=0  F_Comp2_In=off  F_Comp2=0  F_Comp3_In=off  F_Comp3=0  F_Comp4_In=off  F_Comp4=0
      settings: SourceProductName=Target Support Package - STM32 Adapter
  modeWrite : DataStoreWrite  DataStoreName=mode
  wires:
  ONE_PHASE/1 -> modeWrite/1
  1/1 -> Add1/1, Add/2
  PERIOD/1 -> Add1/3, Add/1
  Add/1 -> Set1/1
  ADCConvTime Read/1 -> Product/1
  4/1 -> Product/2
  Product/1 -> Add1/2
  Add1/1 -> Set1/2

== system Multiphase/RepHRTimM/Subsystem ==
  Get : HRTIMERS_Lib/Get  Priority=-1  currentHRTIM=HRTIM1  NbHRTim=1  HRTIM_Name=HRTIM1  M_Used=on  M_Period=on  M_Comp1=off  M_Comp2=off  M_Comp3=off  M_Comp4=off  A_Used=on  A_Period=off  A_Capt1_In=off  A_Capt2_In=off  A_Info=Timer A TA1 and TA2 lines are not configured as input.  A_Comp1=off  A_Comp2=off  A_Comp3=off  A_Comp4=off  B_Used=on  B_Period=off  B_Capt1_In=off  B_Capt2_In=off  B_Info=Timer B TB1 and TB2 lines are not configured as input.  B_Comp1=off  B_Comp2=off  B_Comp3=off  B_Comp4=off  C_Used=on  C_Period=off  C_Capt1_In=off  C_Capt2_In=off  C_Info=Timer C TC1 and TC2 lines are not configured as input.  C_Comp1=off  C_Comp2=off  C_Comp3=off  C_Comp4=off  D_Used=on  D_Period=off  D_Capt1_In=off  D_Capt2_In=off  D_Info=Timer D TD1 and TD2 lines are not configured as input.  D_Comp1=off  D_Comp2=off  D_Comp3=off  D_Comp4=off  E_Used=off  E_Period=off  E_Capt1_In=off  E_Capt2_In=off  E_Info=Timer E is not configured.  E_Comp1=off  E_Comp2=off  E_Comp3=off  E_Comp4=off  F_Used=off  F_Period=off  F_Capt1_In=off  F_Capt2_In=off  F_Info=Timer F is not configured.  F_Comp1=off  F_Comp2=off  F_Comp3=off  F_Comp4=off
      settings: SourceProductName=Target Support Package - STM32 Adapter
  MULTIPHASE_PERIOD : Outport
  wires:
  Get/1 -> MULTIPHASE_PERIOD/1

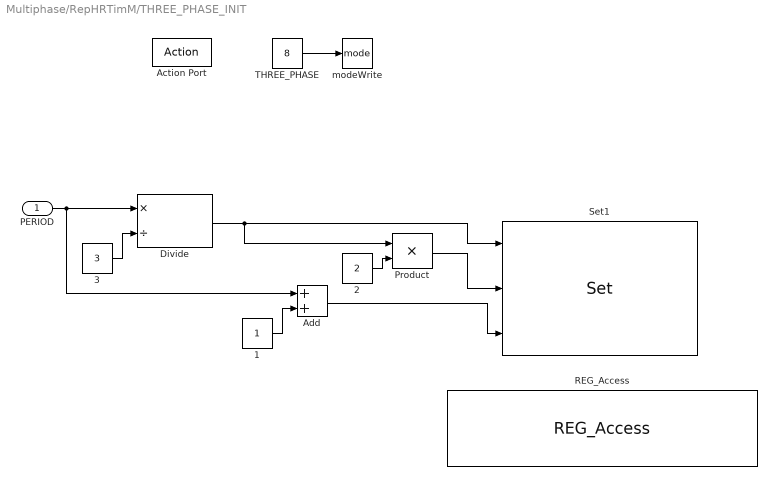
== system Multiphase/RepHRTimM/THREE_PHASE_INIT ==
  PERIOD : Inport
  Action Port : ActionPort  ActionType=case
  1 : Constant  OutDataTypeStr=uint32
  2 : Constant  Value=2  OutDataTypeStr=uint32
  3 : Constant  Value=3  OutDataTypeStr=uint32
  Add : Sum  AccumDataTypeStr=uint32  InputSameDT=on
  Divide : Product  Inputs=*/  OutDataTypeStr=uint32  InputSameDT=on
  Product : Product  OutDataTypeStr=uint32  InputSameDT=on
  REG_Access : REG_Lib/REG_Access  Peripheral=HRTIM1  RegName=sCommonRegs.ADC1R  RegRead=off  RegWrite=on  RegValueIn=off  RegValue=<binary blob, 179 chars, not shown>  RegEqual=on  RegAnd=off  RegOr=off  RegComplement=off  RegComments=Reconfigure ADC triggers for a dummy 4th and 5th conversion  currentPeriph=HRTIM1
      settings: SourceProductName=Target Support Package - STM32 Adapter
  Set1 : HRTIMERS_Lib/Set  currentHRTIM=HRTIM1  NbHRTim=1  HRTIM_Name=HRTIM1  M_Used=on  M_Comp1_In=on  M_Comp1=0  M_Comp2_In=on  M_Comp2=0  M_Comp3_In=on  M_Comp3=0  M_Comp4_In=off  M_Comp4=0  A_Used=on  A_Comp1_In=off  A_Comp1=0  A_Comp2_In=off  A_Comp2=0  A_Comp3_In=off  A_Comp3=0  A_Comp4_In=off  A_Comp4=0  B_Used=on  B_Comp1_In=off  B_Comp1=0  B_Comp2_In=off  B_Comp2=0  B_Comp3_In=off  B_Comp3=0  B_Comp4_In=off  B_Comp4=0  C_Used=on  C_Comp1_In=off  C_Comp1=0  C_Comp2_In=off  C_Comp2=0  C_Comp3_In=off  C_Comp3=0  C_Comp4_In=off  C_Comp4=0  D_Used=on  D_Comp1_In=off  D_Comp1=0  D_Comp2_In=off  D_Comp2=0  D_Comp3_In=off  D_Comp3=0  D_Comp4_In=off  D_Comp4=0  E_Used=off  E_Comp1_In=off  E_Comp1=0  E_Comp2_In=off  E_Comp2=0  E_Comp3_In=off  E_Comp3=0  E_Comp4_In=off  E_Comp4=0  F_Used=off  F_Comp1_In=off  F_Comp1=0  F_Comp2_In=off  F_Comp2=0  F_Comp3_In=off  F_Comp3=0  F_Comp4_In=off  F_Comp4=0
      settings: SourceProductName=Target Support Package - STM32 Adapter
  THREE_PHASE : Constant  Value=8  OutDataTypeStr=uint8
  modeWrite : DataStoreWrite  DataStoreName=mode
  wires:
  THREE_PHASE/1 -> modeWrite/1
  PERIOD/1 -> Add/1, Divide/1
  3/1 -> Divide/2
  Divide/1 -> Product/1, Set1/1
  Product/1 -> Set1/2
  2/1 -> Product/2
  Add/1 -> Set1/3
  1/1 -> Add/2

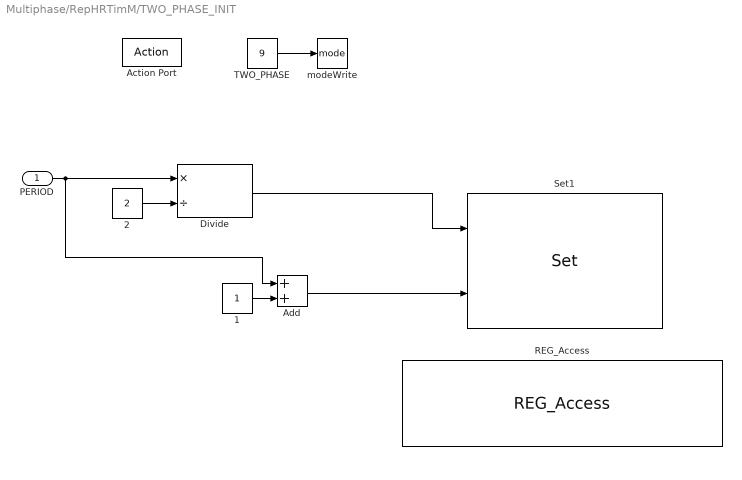
== system Multiphase/RepHRTimM/TWO_PHASE_INIT ==
  PERIOD : Inport
  Action Port : ActionPort  ActionType=case
  1 : Constant  OutDataTypeStr=uint32
  2 : Constant  Value=2  OutDataTypeStr=uint32
  Add : Sum  AccumDataTypeStr=uint32  InputSameDT=on
  Divide : Product  Inputs=*/  OutDataTypeStr=uint32  InputSameDT=on
  REG_Access : REG_Lib/REG_Access  Peripheral=HRTIM1  RegName=sCommonRegs.ADC1R  RegRead=off  RegWrite=on  RegValueIn=off  RegValue=<binary blob, 179 chars, not shown>  RegEqual=on  RegAnd=off  RegOr=off  RegComplement=off  RegComments=Reconfigure ADC triggers for a dummy 3rd, 4th and 5th conversion  currentPeriph=HRTIM1
      settings: SourceProductName=Target Support Package - STM32 Adapter
  Set1 : HRTIMERS_Lib/Set  currentHRTIM=HRTIM1  NbHRTim=1  HRTIM_Name=HRTIM1  M_Used=on  M_Comp1_In=on  M_Comp1=0  M_Comp2_In=on  M_Comp2=0  M_Comp3_In=off  M_Comp3=0  M_Comp4_In=off  M_Comp4=0  A_Used=on  A_Comp1_In=off  A_Comp1=0  A_Comp2_In=off  A_Comp2=0  A_Comp3_In=off  A_Comp3=0  A_Comp4_In=off  A_Comp4=0  B_Used=on  B_Comp1_In=off  B_Comp1=0  B_Comp2_In=off  B_Comp2=0  B_Comp3_In=off  B_Comp3=0  B_Comp4_In=off  B_Comp4=0  C_Used=on  C_Comp1_In=off  C_Comp1=0  C_Comp2_In=off  C_Comp2=0  C_Comp3_In=off  C_Comp3=0  C_Comp4_In=off  C_Comp4=0  D_Used=on  D_Comp1_In=off  D_Comp1=0  D_Comp2_In=off  D_Comp2=0  D_Comp3_In=off  D_Comp3=0  D_Comp4_In=off  D_Comp4=0  E_Used=off  E_Comp1_In=off  E_Comp1=0  E_Comp2_In=off  E_Comp2=0  E_Comp3_In=off  E_Comp3=0  E_Comp4_In=off  E_Comp4=0  F_Used=off  F_Comp1_In=off  F_Comp1=0  F_Comp2_In=off  F_Comp2=0  F_Comp3_In=off  F_Comp3=0  F_Comp4_In=off  F_Comp4=0
      settings: SourceProductName=Target Support Package - STM32 Adapter
  TWO_PHASE : Constant  Value=9  OutDataTypeStr=uint8
  modeWrite : DataStoreWrite  DataStoreName=mode
  wires:
  TWO_PHASE/1 -> modeWrite/1
  PERIOD/1 -> Add/1, Divide/1
  2/1 -> Divide/2
  Divide/1 -> Set1/1
  1/1 -> Add/2
  Add/1 -> Set1/2

== system Multiphase/modeSelect/BURST ==
  BURST : ActionPort  ActionType=case
  FIVE_PHASE_INIT : Constant  Value=0  OutDataTypeStr=uint8
  modeWrite : DataStoreWrite  DataStoreName=mode
  wires:
  FIVE_PHASE_INIT/1 -> modeWrite/1

== system Multiphase/modeSelect/FAULT ==
  FAULT : ActionPort  ActionType=case
  FIVE_PHASE_INIT : Constant  Value=0  OutDataTypeStr=uint8
  Start : HRTIMERS_Lib/Start  currentHRTIM=HRTIM1  NbHRTim=1  HRTIM_Name=HRTIM1  TA1_Start=off  TA2_Start=on  TB1_Start=on  TB2_Start=off  TC1_Start=off  TC2_Start=on  TD1_Start=on  TD2_Start=on  TE1_Start=off  TE2_Start=off  TF1_Start=off  TF2_Start=off
      settings: SourceProductName=Target Support Package - STM32 Adapter
  modeWrite : DataStoreWrite  DataStoreName=mode
  wires:
  FIVE_PHASE_INIT/1 -> modeWrite/1

== system Multiphase/modeSelect/FIVE_PHASE ==
  FIVE_PHASE : ActionPort  ActionType=case
  FOUR_PHASE_INIT : Constant  OutDataTypeStr=uint8
  modeWrite : DataStoreWrite  DataStoreName=mode
  wires:
  FOUR_PHASE_INIT/1 -> modeWrite/1

== system Multiphase/modeSelect/FOUR_PHASE ==
  FOUR_PHASE : ActionPort  ActionType=case
  THREE_PHASE_INIT : Constant  Value=2  OutDataTypeStr=uint8
  modeWrite : DataStoreWrite  DataStoreName=mode
  wires:
  THREE_PHASE_INIT/1 -> modeWrite/1

== system Multiphase/modeSelect/ONE_PHASE ==
  ONE_PHASE : ActionPort  ActionType=case
  BURST_INIT : Constant  Value=5  OutDataTypeStr=uint8
  modeWrite : DataStoreWrite  DataStoreName=mode
  wires:
  BURST_INIT/1 -> modeWrite/1

== system Multiphase/modeSelect/THREE_PHASE ==
  THREE_PHASE : ActionPort  ActionType=case
  TWO_PHASE_INIT : Constant  Value=3  OutDataTypeStr=uint8
  modeWrite : DataStoreWrite  DataStoreName=mode
  wires:
  TWO_PHASE_INIT/1 -> modeWrite/1

== system Multiphase/modeSelect/TWO_PHASE ==
  TWO_PHASE : ActionPort  ActionType=case
  ONE_PHASE_INIT : Constant  Value=4  OutDataTypeStr=uint8
  modeWrite : DataStoreWrite  DataStoreName=mode
  wires:
  ONE_PHASE_INIT/1 -> modeWrite/1
